simulink library "CellsLib"  (Simulink 7.7)
settings: Solver=ode45  SolverMode=SingleTasking  StartTime=0.0  StopTime=10.0  RelTol=1e-3
libraries: CompartmentsLib x26, CurrentsLib x23, SpikingLib x9, SynapsesLib x7, WaveformsLib x1, BasicSpikingElementsLib x1, SpikeToWavesLib x1, RateBasedLib x1
settings Model: Creator=jpalma  LastModifiedBy=jpalma

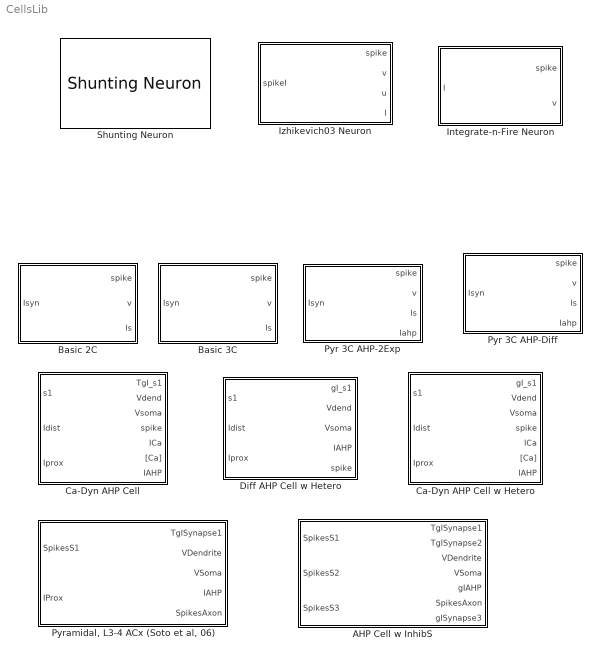
== system CellsLib ==
  AHP Cell w InhibS : Subsystem  mask{PSoma1=[1 -65 45 50 16 -100 0.1 -65 0.28 0.1 0.15], PDend2=[1 -65 0.03 -65 0.28 0.06 0.4], PDend3=[1 -65 0.03 -65 0.28 0.06 0.5], PfAHP=[-65 0.8 0.1 2.0], PmAHP=[-97 0.04 18 164], PsAHP=[-100 0.02 225 2200], PAmpa=[0 2 0.76 6.5], PAmpa2=[0 0.2 0.76 6.5], PGaba=[-90 2 0.76 6.5], spikeThreshold=10}
      mask prompts: PSoma1 "Soma Params [C1 V01 gNa1 ENa1 gK1 EK1 gL1 EL1 gA1 d1 L1]"; PDend2 "Prox Dend Params [C2 V02 gL2 EL2 gA2 d2 L2]"; PDend3 "Dist Dend Params [C3 V03 gL3 EL3 gA3 d3 L3]"; PfAHP "fAHP Params [EfAHP gfAHP RTfAHP FTfAHP]"; PmAHP "mAHP Params [EmAHP gmAHP RTmAHP FTmAHP]"; PsAHP "sAHP Params [EsAHP gsAHP RTsAHP FTsAHP]"; PAmpa "AMPA Params [EAmpa gAmpa RTampa FTampa]"; PAmpa2 "AMPA2 Params [EAmpa2 gAmpa2 RTampa2 FTampa2]"; PGaba "GABA Params [EGaba gGaba RTgaba FTgaba]"; spikeThreshold "Spike Detection Voltage Threshold"
      mask help: Author: Jesse Palma
      mask Help: Author: Jesse Palma
      mask Display: image(imread('../Libs/icons/Cell.jpg'),'center');
  Basic 2C : Subsystem  mask{PSoma1=[1 -65 45 50 16 -100 0.1 -65 0.28 0.1 0.15], PDend2=[1 -65 0.03 -65 0.28 0.06 0.4], spikeThreshold=10}
      mask prompts: PSoma1 "Soma Params [C1 V01 gNa1 ENa1 gK1 EK1 gL1 EL1 gA1 d1 L1]"; PDend2 "Dend Params [C2 V02 gL2 EL2 gA2 d2 L2]"; spikeThreshold "Spike Detection Voltage Threshold"
      mask help: Author: Jesse Palma
      settings: AttributesFormatString=%<AncestorBlock>
      mask Help: Author: Jesse Palma
      mask Display: image(imread('../Libs/icons/Cell.jpg'),'center');
  Basic 3C : Subsystem  mask{PSoma1=[1 -65 45 50 16 -100 0.1 -65 0.28 0.1 0.15], PDend2=[1 -65 0.03 -65 0.28 0.06 0.4], PDend3=[1 -65 0.03 -65 0.28 0.06 0.5], spikeThreshold=10}
      mask prompts: PSoma1 "Soma Params [C1 V01 gNa1 ENa1 gK1 EK1 gL1 EL1 gA1 d1 L1]"; PDend2 "Prox Dend Params [C2 V02 gL2 EL2 gA2 d2 L2]"; PDend3 "Dist Dend Params [C3 V03 gL3 EL3 gA3 d3 L3]"; spikeThreshold "Spike Detection Voltage Threshold"
      mask help: Author: Jesse Palma
      settings: AttributesFormatString=%<AncestorBlock>
      mask Help: Author: Jesse Palma
      mask Display: image(imread('../Libs/icons/Cell.jpg'),'center');
  Ca-Dyn AHP Cell : Subsystem  mask{C1=1, V01=-65, spikeThreshold=10, gA1=0.28, d1=0.1, L1=0.15, gNa1=45, ENa1=50, gK1=16, EK1=-100, gL1=0.1, EL1=-65, gBK1=4.0, EBK1=-65, gKA=0.5, EKA=-100, gSK1=0.08, ESK1=-97, gKM=0.1, EKM=-97, gsAHP1=0.025, EsAHP1=-100, gvsAHP=0.1, EvsAHP=-100, C2=1, V02=-65, gL2=0.03, EL2=-65, gA2=0.28, d2=0.06, L2=0.4, C3=1, V03=-65, gL3=0.03, EL3=-65, gA3=0.28, d3=0.06, L3=0.5, gampa=1, Eampa=0, RTampa=0.76, FTampa=6.5}
      mask prompts: C1 "Capacitance"; V01 "Initial Voltage"; spikeThreshold "Spike Detection Voltage Threshold"; gA1 "Axial Conductance"; d1 "Diameter"; L1 "Length"; gNa1 "Sodium Conductance"; ENa1 "Sodium Equilibrium Potential"; gK1 "Potassium Conductance"; EK1 "Potassium Equilibrium Potential"; gL1 "Leak Conductance"; EL1 "Leak Equilibrium Potential"; gBK1 "BK Conductance"; EBK1 "BK Equilibrium Potential"; gKA "K(A) Conductance"; EKA "K(A) Equilibrium Potential"; gSK1 "SK Conductance"; ESK1 "SK Equilibrium Potential"; gKM "K(M) Conductance"; EKM "K(M) Equilibrium Potential"; gsAHP1 "sAHP Conductance"; EsAHP1 "sAHP Equilibrium Potential"; gvsAHP "V sAHP Conductance"; EvsAHP "V sAHP Equilibrium Potential"; C2 "Capacitance"; V02 "Initial Voltage"; gL2 "Leak Conductance"; EL2 "Leak Equilibrium Potential"; gA2 "Axial Conductance"; d2 "Diameter"; L2 "Length"; C3 "Capacitance"; V03 "Initial Voltage"; gL3 "Leak Conductance"; EL3 "Leak Equilibrium Potential"; gA3 "Axial Conductance"; d3 "Diameter"; L3 "Length"; gampa "Conductance"; Eampa "Equilibrium Potential"; RTampa "Rise Time"; FTampa "Fall Time"
      mask help: Author: Jesse Palma
      mask Help: Author: Jesse Palma
      mask TabNameString: Soma Base, Soma Base, Soma Base, Soma Base, Soma Base, Soma Base,Currents,Currents,Currents,Currents,Currents,Currents,AHP,AHP,AHP,AHP,AHP,AHP,AHP,AHP,AHP,AHP,AHP,AHP,Prox,Prox,Prox,Prox,Prox,Prox,Prox,Dist,Dist,Dist,Dist,Dist,Dist,Dist,AMPA,AMPA,AMPA,AMPA
      mask Display: image(imread('../Libs/icons/Cell.jpg'),'center');
  Ca-Dyn AHP Cell w Hetero : Subsystem  mask{C1=1, V01=-65, spikeThreshold=10, gA1=0.28, d1=0.1, L1=0.15, gNa1=45, ENa1=50, gK1=16, EK1=-100, gL1=0.1, EL1=-65, gBK1=4.0, EBK1=-65, gKA=0.5, EKA=-100, gSK1=0.08, ESK1=-97, gKM=0.1, EKM=-97, gsAHP1=0.025, EsAHP1=-100, gvsAHP=0.1, EvsAHP=-100, C2=1, V02=-65, gL2=0.03, EL2=-65, gA2=0.28, d2=0.06, L2=0.4, C3=1, V03=-65, gL3=0.03, EL3=-65, gA3=0.28, d3=0.06, L3=0.5, gampa=1, Eampa=0, RTampa=0.76, FTampa=6.5}
      mask prompts: C1 "Capacitance"; V01 "Initial Voltage"; spikeThreshold "Spike Detection Voltage Threshold"; gA1 "Axial Conductance"; d1 "Diameter"; L1 "Length"; gNa1 "Sodium Conductance"; ENa1 "Sodium Equilibrium Potential"; gK1 "Potassium Conductance"; EK1 "Potassium Equilibrium Potential"; gL1 "Leak Conductance"; EL1 "Leak Equilibrium Potential"; gBK1 "BK Conductance"; EBK1 "BK Equilibrium Potential"; gKA "K(A) Conductance"; EKA "K(A) Equilibrium Potential"; gSK1 "SK Conductance"; ESK1 "SK Equilibrium Potential"; gKM "K(M) Conductance"; EKM "K(M) Equilibrium Potential"; gsAHP1 "sAHP Conductance"; EsAHP1 "sAHP Equilibrium Potential"; gvsAHP "V sAHP Conductance"; EvsAHP "V sAHP Equilibrium Potential"; C2 "Capacitance"; V02 "Initial Voltage"; gL2 "Leak Conductance"; EL2 "Leak Equilibrium Potential"; gA2 "Axial Conductance"; d2 "Diameter"; L2 "Length"; C3 "Capacitance"; V03 "Initial Voltage"; gL3 "Leak Conductance"; EL3 "Leak Equilibrium Potential"; gA3 "Axial Conductance"; d3 "Diameter"; L3 "Length"; gampa "Conductance"; Eampa "Equilibrium Potential"; RTampa "Rise Time"; FTampa "Fall Time"
      mask help: Author: Jesse Palma
      mask Help: Author: Jesse Palma
      mask TabNameString: Soma Base, Soma Base, Soma Base, Soma Base, Soma Base, Soma Base,Currents,Currents,Currents,Currents,Currents,Currents,AHP,AHP,AHP,AHP,AHP,AHP,AHP,AHP,AHP,AHP,AHP,AHP,Prox,Prox,Prox,Prox,Prox,Prox,Prox,Dist,Dist,Dist,Dist,Dist,Dist,Dist,AMPA,AMPA,AMPA,AMPA
      mask Display: image(imread('../Libs/icons/Cell.jpg'),'center');
  "Diff AHP Cell w Hetero " : Subsystem  mask{PSoma1=[1 -65 45 50 16 -100 0.1 -65 0.28 0.1 0.15], PDend2=[1 -65 0.03 -65 0.28 0.06 0.4], PDend3=[1 -65 0.03 -65 0.28 0.06 0.5], PfAHP=[-65 0.8 0.1 2.0], PmAHP=[-97 0.04 18 164], PsAHP=[-100 0.02 225 2200], PAmpa=[0 1 0.76 6.5], spikeThreshold=10}
      mask prompts: PSoma1 "Soma Params [C1 V01 gNa1 ENa1 gK1 EK1 gL1 EL1 gA1 d1 L1]"; PDend2 "Prox Dend Params [C2 V02 gL2 EL2 gA2 d2 L2]"; PDend3 "Dist Dend Params [C3 V03 gL3 EL3 gA3 d3 L3]"; PfAHP "fAHP Params [EfAHP gfAHP RTfAHP FTfAHP]"; PmAHP "mAHP Params [EmAHP gmAHP RTmAHP FTmAHP]"; PsAHP "sAHP Params [EsAHP gsAHP RTsAHP FTsAHP]"; PAmpa "AMPA Params [EAmpa gAmpa RTampa FTampa]"; spikeThreshold "Spike Detection Voltage Threshold"
      mask help: Author: Jesse Palma
      mask Help: Author: Jesse Palma
      mask Display: image(imread('../Libs/icons/Cell.jpg'),'center');
  Integrate-n-Fire Neuron : Subsystem  mask{A=0.05, SpikeThreshold=1}
      mask prompts: A "Decay Rate"; SpikeThreshold "Spike Threshold"
      mask help: Author: Jesse Palma
      mask Help: Author: Jesse Palma
      mask Display: image(imread('IntFire.JPG'),'center');
  Izhikevich03 Neuron : Subsystem
      mask Description: Author: Jesse Palma
      mask Help: Author: Jesse Palma
      mask Display: image(imread('../Libs/icons/Izhik.jpg'),'center');
  Pyr 3C AHP-2Exp : Subsystem  mask{PSoma1=[1 -65 45 50 16 -100 0.1 -65 0.28 0.1 0.15], PDend2=[1 -65 0.03 -65 0.28 0.06 0.4], PDend3=[1 -65 0.03 -65 0.28 0.06 0.5], PfAHP=[-65 0.8 0.1 2.0], PmAHP=[-97 0.04 18 164], PsAHP=[-100 0.02 225 2200], spikeThreshold=10}
      mask prompts: PSoma1 "Soma Params [C1 V01 gNa1 ENa1 gK1 EK1 gL1 EL1 gA1 d1 L1]"; PDend2 "Prox Dend Params [C2 V02 gL2 EL2 gA2 d2 L2]"; PDend3 "Dist Dend Params [C3 V03 gL3 EL3 gA3 d3 L3]"; PfAHP "fAHP Params [EfAHP gfAHP RTfAHP FTfAHP]"; PmAHP "mAHP Params [EmAHP gmAHP RTmAHP FTmAHP]"; PsAHP "sAHP Params [EsAHP gsAHP RTsAHP FTsAHP]"; spikeThreshold "Spike Detection Voltage Threshold"
      mask help: Author: Jesse Palma
      mask Help: Author: Jesse Palma
      mask Display: image(imread('../Libs/icons/Cell.jpg'),'center');
  Pyr 3C AHP-Diff : Subsystem  mask{PSoma1=[1 -65 45 50 16 -100 0.1 -65 0.28 0.1 0.15], PDend2=[1 -65 0.03 -65 0.28 0.06 0.4], PDend3=[1 -65 0.03 -65 0.28 0.06 0.5], PfAHP=[-65 0.8 0.1 2.0], PmAHP=[-97 0.04 18 164], PsAHP=[-100 0.02 225 2200], spikeThreshold=10}
      mask prompts: PSoma1 "Soma Params [C1 V01 gNa1 ENa1 gK1 EK1 gL1 EL1 gA1 d1 L1]"; PDend2 "Prox Dend Params [C2 V02 gL2 EL2 gA2 d2 L2]"; PDend3 "Dist Dend Params [C3 V03 gL3 EL3 gA3 d3 L3]"; PfAHP "fAHP Params [EfAHP gfAHP RTfAHP FTfAHP]"; PmAHP "mAHP Params [EmAHP gmAHP RTmAHP FTmAHP]"; PsAHP "sAHP Params [EsAHP gsAHP RTsAHP FTsAHP]"; spikeThreshold "Spike Detection Voltage Threshold"
      mask help: Author: Jesse Palma
      settings: AttributesFormatString=%<AncestorBlock>
      mask Help: Author: Jesse Palma
      mask Display: image(imread('../Libs/icons/Cell.jpg'),'center');
  "Pyramidal, L3-4 ACx (Soto et al, 06)" : Subsystem  mask{PSoma1=[1 -65 45 50 16 -100 0.1 -65 0.28 0.1 0.15], PDend2=[1 -65 0.03 -65 0.28 0.06 0.4], PDend3=[1 -65 0.03 -65 0.28 0.06 0.5], PfAHP=[-65 0.8 0.1 2.0], PmAHP=[-97 0.04 18 164], PsAHP=[-100 0.02 225 2200], PAmpa=[0 1 0.76 6.5], spikeThreshold=10}
      mask prompts: PSoma1 "Soma Params [C1 V01 gNa1 ENa1 gK1 EK1 gL1 EL1 gA1 d1 L1]"; PDend2 "Prox Dend Params [C2 V02 gL2 EL2 gA2 d2 L2]"; PDend3 "Dist Dend Params [C3 V03 gL3 EL3 gA3 d3 L3]"; PfAHP "fAHP Params [EfAHP gfAHP RTfAHP FTfAHP]"; PmAHP "mAHP Params [EmAHP gmAHP RTmAHP FTmAHP]"; PsAHP "sAHP Params [EsAHP gsAHP RTsAHP FTsAHP]"; PAmpa "AMPA Params [EAmpa gAmpa RTampa FTampa]"; spikeThreshold "Spike Detection Voltage Threshold"
      mask help: Author: Jesse Palma
      mask Help: Author: Jesse Palma
      mask Display: image(imread('../Libs/icons/Cell.jpg'),'center');
  Shunting Neuron : RateBasedLib/Shunting Neuron  SystemSampleTime=-1  A=0.1  B=1  tau=1

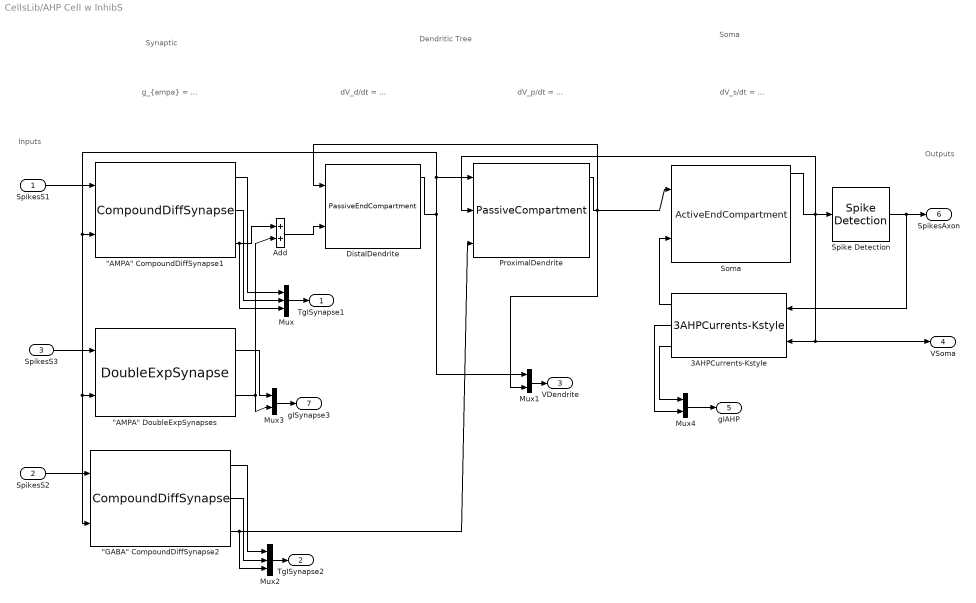
== system CellsLib/AHP Cell w InhibS ==
  note: Inputs
  note: Outputs
  note: Soma
  note: Dendritic Tree
  note: Synaptic
  note: g_{ampa} = ...
  note: dV_s/dt = ...
  note: dV_p/dt = ...
  note: dV_d/dt = ...
  SpikesS1 : Inport
  SpikesS2 : Inport  Port=2
  SpikesS3 : Inport  Port=3
  "\"AMPA\" CompoundDiffSynapse1" : SynapsesLib/CompoundDiffSynapse  SystemSampleTime=-1  EZ=PAmpa(1)  gZ=PAmpa(2)  tauRZ=PAmpa(3)  tauFZ=PAmpa(4)
  "\"AMPA\" DoubleExpSynapses" : SynapsesLib/DoubleExpSynapse  SystemSampleTime=-1  EZ=PAmpa2(1)  gZ=PAmpa2(2)  tauRZ=PAmpa2(3)  tauFZ=PAmpa2(4)
  "\"GABA\" CompoundDiffSynapse2" : SynapsesLib/CompoundDiffSynapse  SystemSampleTime=-1  EZ=PGaba(1)  gZ=PGaba(2)  tauRZ=PGaba(3)  tauFZ=PGaba(4)
  3AHPCurrents-Kstyle : CurrentsLib/3AHPCurrents-Kstyle  SystemSampleTime=-1  EfAHP=PfAHP(1)  gfAHP=PfAHP(2)  tauRfAHP=PfAHP(3)  tauFfAHP=PfAHP(4)  EmAHP=PmAHP(1)  gmAHP=PmAHP(2)  tauRmAHP=PmAHP(3)  tauFmAHP=PmAHP(4)  EsAHP=PsAHP(1)  gsAHP=PsAHP(2)  tauRsAHP=PsAHP(3)  tauFsAHP=PsAHP(4)
  Add : Sum
  DistalDendrite : CompartmentsLib/PassiveEndCompartment  SystemSampleTime=-1  C=PDend3(1)  V0=PDend3(2)  gA=PDend3(5)  d=PDend3(6)  L=PDend3(7)  gL=PDend3(3)  EL=PDend3(4)
  Mux : Mux  Inputs=3
  Mux1 : Mux  Inputs=2
  Mux2 : Mux  Inputs=3
  Mux3 : Mux  Inputs=2
  Mux4 : Mux  Inputs=2
  ProximalDendrite : CompartmentsLib/PassiveCompartment  SystemSampleTime=-1  C=PDend2(1)  V0=PDend2(2)  gA=PDend2(5)  d=PDend2(6)  L=PDend2(7)  gL=PDend2(3)  EL=PDend2(4)
  Soma : CompartmentsLib/ActiveEndCompartment  SystemSampleTime=-1  C=PSoma1(1)  V0=PSoma1(2)  gA=PSoma1(9)  d=PSoma1(10)  L=PSoma1(11)  gNa=PSoma1(3)  ENa=PSoma1(4)  gK=PSoma1(5)  EK=PSoma1(6)  gL=PSoma1(7)  EL=PSoma1(8)
  Spike Detection : SpikingLib/Spike Detection  SystemSampleTime=-1  SpikeVoltageThreshold=spikeThreshold
  TgISynapse1 : Outport
  TgISynapse2 : Outport  Port=2
  VDendrite : Outport  Port=3
  VSoma : Outport  Port=4
  gIAHP : Outport  Port=5
  SpikesAxon : Outport  Port=6
  gISynapse3 : Outport  Port=7
  wires:
  Mux1/1 -> VDendrite/1
  "\"AMPA\" CompoundDiffSynapse1"/1 -> Mux/1
  Mux/1 -> TgISynapse1/1
  "\"AMPA\" CompoundDiffSynapse1"/3 -> Mux/3, Add/1
  "\"AMPA\" CompoundDiffSynapse1"/2 -> Mux/2
  SpikesS1/1 -> "\"AMPA\" CompoundDiffSynapse1"/1
  Spike Detection/1 -> 3AHPCurrents-Kstyle/1, SpikesAxon/1
  Soma/1 -> ProximalDendrite/2, 3AHPCurrents-Kstyle/2, VSoma/1, Spike Detection/1
  ProximalDendrite/1 -> Mux1/2, Soma/1, DistalDendrite/1
  DistalDendrite/1 -> Mux1/1, ProximalDendrite/1, "\"AMPA\" CompoundDiffSynapse1"/2, "\"GABA\" CompoundDiffSynapse2"/2, "\"AMPA\" DoubleExpSynapses"/2
  SpikesS2/1 -> "\"GABA\" CompoundDiffSynapse2"/1
  Mux2/1 -> TgISynapse2/1
  "\"GABA\" CompoundDiffSynapse2"/1 -> Mux2/1
  "\"GABA\" CompoundDiffSynapse2"/2 -> Mux2/2
  "\"GABA\" CompoundDiffSynapse2"/3 -> ProximalDendrite/3, Mux2/3
  3AHPCurrents-Kstyle/1 -> Soma/2
  SpikesS3/1 -> "\"AMPA\" DoubleExpSynapses"/1
  Mux3/1 -> gISynapse3/1
  "\"AMPA\" DoubleExpSynapses"/1 -> Mux3/1
  "\"AMPA\" DoubleExpSynapses"/2 -> Mux3/2, Add/2
  Add/1 -> DistalDendrite/2
  Mux4/1 -> gIAHP/1
  3AHPCurrents-Kstyle/3 -> Mux4/1
  3AHPCurrents-Kstyle/2 -> Mux4/2

== system CellsLib/Basic 2C ==
  note: Soma
  note: dV_s/dt = ...
  note: dV_d/dt = ...
  note: Dendrite
  Isyn : Inport
  Bus Creator : BusCreator  Inputs=2
  Bus Creator1 : BusCreator
  Bus Selector : BusSelector  OutputSignals=signal1,signal2
  DistalDendrite : CompartmentsLib/PassiveEndCompartment  SystemSampleTime=-1  C=PDend2(1)  V0=PDend2(2)  gA=PDend2(5)  d=PDend2(6)  L=PDend2(7)  gL=PDend2(3)  EL=PDend2(4)
  Soma : CompartmentsLib/ActiveEndCompartment  SystemSampleTime=-1  C=PSoma1(1)  V0=PSoma1(2)  gA=PSoma1(9)  d=PSoma1(10)  L=PSoma1(11)  gNa=PSoma1(3)  ENa=PSoma1(4)  gK=PSoma1(5)  EK=PSoma1(6)  gL=PSoma1(7)  EL=PSoma1(8)
  Spike Detection : SpikingLib/Spike Detection  SystemSampleTime=-1  SpikeVoltageThreshold=spikeThreshold
  spike : Outport
  v : Outport  Port=2
  Is : Outport  Port=3
  wires:
  DistalDendrite/1 -> Soma/1, Bus Creator/1
  Soma/1 -> Spike Detection/1, DistalDendrite/1, Bus Creator/2
  Spike Detection/1 -> spike/1
  Isyn/1 -> Bus Selector/1
  Soma/2 -> Bus Creator1/1
  Soma/3 -> Bus Creator1/2
  Soma/4 -> Bus Creator1/3
  Soma/5 -> Bus Creator1/4
  Bus Creator1/1 -> Is/1
  Bus Selector/2 -> Soma/2
  Bus Creator/1 -> v/1
  Bus Selector/1 -> DistalDendrite/2

== system CellsLib/Basic 3C ==
  note: dV_d/dt = ...
  note: dV_p/dt = ...
  note: dV_s/dt = ...
  note: Dendritic Tree
  note: Soma
  Isyn : Inport
  Demux : Demux  Outputs=3
  DistalDendrite : CompartmentsLib/PassiveEndCompartment  SystemSampleTime=-1  C=PDend3(1)  V0=PDend3(2)  gA=PDend3(5)  d=PDend3(6)  L=PDend3(7)  gL=PDend3(3)  EL=PDend3(4)
  Mux : Mux
  Mux1 : Mux  Inputs=3
  ProximalDendrite : CompartmentsLib/PassiveCompartment  SystemSampleTime=-1  C=PDend2(1)  V0=PDend2(2)  gA=PDend2(5)  d=PDend2(6)  L=PDend2(7)  gL=PDend2(3)  EL=PDend2(4)
  Soma : CompartmentsLib/ActiveEndCompartment  SystemSampleTime=-1  C=PSoma1(1)  V0=PSoma1(2)  gA=PSoma1(9)  d=PSoma1(10)  L=PSoma1(11)  gNa=PSoma1(3)  ENa=PSoma1(4)  gK=PSoma1(5)  EK=PSoma1(6)  gL=PSoma1(7)  EL=PSoma1(8)
  Spike Detection : SpikingLib/Spike Detection  SystemSampleTime=-1  SpikeVoltageThreshold=spikeThreshold
  spike : Outport
  v : Outport  Port=2
  Is : Outport  Port=3
  wires:
  Mux1/1 -> v/1
  Demux/3 -> Soma/2
  Demux/2 -> ProximalDendrite/3
  Mux/1 -> Is/1
  Soma/5 -> Mux/4
  Soma/4 -> Mux/3
  Soma/3 -> Mux/2
  Soma/2 -> Mux/1
  Demux/1 -> DistalDendrite/2
  Isyn/1 -> Demux/1
  ProximalDendrite/1 -> Mux1/2, DistalDendrite/1, Soma/1
  Spike Detection/1 -> spike/1
  Soma/1 -> Mux1/3, ProximalDendrite/2, Spike Detection/1
  DistalDendrite/1 -> Mux1/1, ProximalDendrite/1

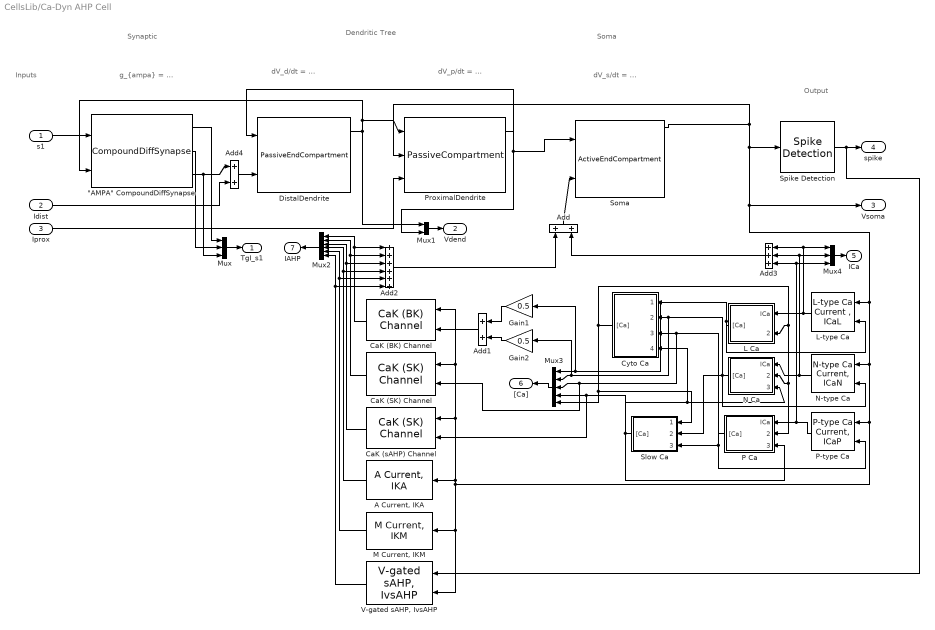
== system CellsLib/Ca-Dyn AHP Cell ==
  note: Inputs
  note: Output
  note: Soma
  note: Dendritic Tree
  note: Synaptic
  note: g_{ampa} = ...
  note: dV_s/dt = ...
  note: dV_p/dt = ...
  note: dV_d/dt = ...
  s1 : Inport
  Idist : Inport  Port=2
  Iprox : Inport  Port=3
  "\"AMPA\" CompoundDiffSynapse" : SynapsesLib/CompoundDiffSynapse  SystemSampleTime=-1  EZ=Eampa  gZ=gampa  tauRZ=RTampa  tauFZ=FTampa
  "A Current, IKA" : CurrentsLib/A Current, IKA  SystemSampleTime=-1  EKA=EKA  gKA=gKA  m_a=KAm_alpha  m_b=KAm_beta  h_a=KAh_alpha  h_b=KAh_beta
  Add : Sum
  Add1 : Sum
  Add2 : Sum  Inputs=++++++
  Add3 : Sum  Inputs=+++
  Add4 : Sum
  CaK (BK) Channel : CurrentsLib/CaK (BK) Channel  SystemSampleTime=-1  EBK=EBK1  gBK=gBK1
  CaK (SK) Channel : CurrentsLib/CaK (SK) Channel  SystemSampleTime=-1  ESK=ESK1  gSK=gSK1
  CaK (sAHP) Channel : CurrentsLib/CaK (SK) Channel  SystemSampleTime=-1  ESK=EsAHP1  gSK=gsAHP1
  Cyto Ca : Subsystem  mask{tauDiff1=800, tauDiff4=3600, tauA=80, caRest=1*10^(-6)}
      mask prompts: tauDiff1 "Diffusion Time Constant, tauDiff1"; tauDiff4 "Diffusion Time Constant, tauDiff4"; tauA "Recovery Time Constant, tauA"; caRest "Calcium Rest Concentration, caRest"
  DistalDendrite : CompartmentsLib/PassiveEndCompartment  SystemSampleTime=-1  C=C3  V0=V03  gA=gA3  d=d3  L=L3  gL=gL3  EL=EL3
  Gain1 : Gain  Gain=0.5
  Gain2 : Gain  Gain=0.5
  L Ca : Subsystem  mask{f=10000/(69843), d=800, a=1/120}
  L-type Ca : CurrentsLib/L-type Ca Current , ICaL  SystemSampleTime=-1  ECaL=130  gCaL=0.00006  m_e=caLm_infin2  m_t=cam_tau2  h_e=caLh_infin2  h_t=cah_tau2
  "M Current, IKM" : CurrentsLib/M Current, IKM  SystemSampleTime=-1  EK=EKM  gK=gKM  m_a=kMm_alpha  m_b=kMm_beta
  Mux : Mux  Inputs=3
  Mux1 : Mux  Inputs=2
  Mux2 : Mux  Inputs=6
  Mux3 : Mux  Inputs=5
  Mux4 : Mux  Inputs=3
  N Ca : Subsystem  mask{f=10000/(69843), d1=800, d2=3600, a=1/360}
  N-type Ca : CurrentsLib/N-type Ca Current, ICaN  SystemSampleTime=-1  ECaN=130  gCaN=0.00005  m_e=caNm_infin2  m_t=cam_tau2  h_e=caNh_infin2  h_t=cah_tau2
  P Ca : Subsystem  mask{f=10000/(69843), d1=800, d2=3600, a=1/60}
  P-type Ca : CurrentsLib/P-type Ca Current, ICaP  SystemSampleTime=-1  ECaP=130  gCaP=0.00009  m_e=caPm_infin2  m_t=cam_tau2  h_e=caPh_infin2  h_t=cah_tau2
  ProximalDendrite : CompartmentsLib/PassiveCompartment  SystemSampleTime=-1  C=C2  V0=V02  gA=gA2  d=d2  L=L2  gL=gL2  EL=EL2
  Slow Ca : Subsystem  mask{tauDiff1=3600, tauDiff2=3600, tauDiff3=3600}
      mask prompts: tauDiff1 "Diffusion Time Constant, tauDiff1"; tauDiff2 "Diffusion Time Constant, tauDiff2"; tauDiff3 "Diffusion Time Constant, tauDiff3"
  Soma : CompartmentsLib/ActiveEndCompartment  SystemSampleTime=-1  C=C1  V0=V01  gA=gA1  d=d1  L=L1  gNa=gNa1  ENa=ENa1  gK=gK1  EK=EK1  gL=gL1  EL=EL1
  Spike Detection : SpikingLib/Spike Detection  SystemSampleTime=-1  SpikeVoltageThreshold=spikeThreshold
  "V-gated sAHP, IvsAHP" : CurrentsLib/V-gated sAHP, IvsAHP  SystemSampleTime=-1  EvsAHP=EvsAHP  gvsAHP=gvsAHP  RvsAHP=225  FvsAHP=2400
  TgI_s1 : Outport
  Vdend : Outport  Port=2
  Vsoma : Outport  Port=3
  spike : Outport  Port=4
  ICa : Outport  Port=5
  "[Ca]" : Outport  Port=6
  IAHP : Outport  Port=7
  wires:
  Mux1/1 -> Vdend/1
  "\"AMPA\" CompoundDiffSynapse"/1 -> Mux/1
  Mux/1 -> TgI_s1/1
  "\"AMPA\" CompoundDiffSynapse"/3 -> Mux/3, Add4/1
  Iprox/1 -> ProximalDendrite/3
  "\"AMPA\" CompoundDiffSynapse"/2 -> Mux/2
  s1/1 -> "\"AMPA\" CompoundDiffSynapse"/1
  Spike Detection/1 -> spike/1, "V-gated sAHP, IvsAHP"/1
  ProximalDendrite/1 -> Mux1/2, Soma/1, DistalDendrite/1
  DistalDendrite/1 -> Mux1/1, ProximalDendrite/1, "\"AMPA\" CompoundDiffSynapse"/2
  L-type Ca/1 -> L Ca/1(ICa), Add3/1, Mux4/1
  P-type Ca/1 -> P Ca/1(ICa), Add3/3, Mux4/3
  L Ca/1("[Ca]") -> Mux3/1, Gain1/1, Cyto Ca/1(AdjCa1), L-type Ca/2
  N Ca/1("[Ca]") -> N-type Ca/2, Slow Ca/2(AdjCa2), Mux3/2, Gain2/1, Cyto Ca/2(AdjCa2)
  P Ca/1("[Ca]") -> P-type Ca/2, Slow Ca/3(AdjCa3), Cyto Ca/3(AdjCa3), Mux3/3, CaK (SK) Channel/2
  Mux3/1 -> "[Ca]"/1
  CaK (SK) Channel/1 -> Add2/2, Mux2/2
  CaK (sAHP) Channel/1 -> Add2/3, Mux2/3
  Soma/1 -> Vsoma/1, L-type Ca/1, N-type Ca/1, P-type Ca/1, CaK (BK) Channel/1, CaK (SK) Channel/1, CaK (sAHP) Channel/1, "V-gated sAHP, IvsAHP"/2, "M Current, IKM"/1, "A Current, IKA"/1, Spike Detection/1, ProximalDendrite/2
  Add/1 -> Soma/2
  Cyto Ca/1("[Ca]") -> L Ca/2(AdjCa), N Ca/2(AdjCa1), P Ca/2(AdjCa1), Slow Ca/1(AdjCa1), Mux3/5
  Slow Ca/1("[Ca]") -> Mux3/4, CaK (sAHP) Channel/2, P Ca/3(AdjCa2), N Ca/3(AdjCa2), Cyto Ca/4(AdjCa4)
  N-type Ca/1 -> N Ca/1(ICa), Add3/2, Mux4/2
  Gain1/1 -> Add1/1
  Gain2/1 -> Add1/2
  Add1/1 -> CaK (BK) Channel/2
  CaK (BK) Channel/1 -> Add2/1, Mux2/1
  Add2/1 -> Add/1
  Add3/1 -> Add/2
  Mux2/1 -> IAHP/1
  Mux4/1 -> ICa/1
  "A Current, IKA"/1 -> Add2/4, Mux2/4
  "M Current, IKM"/1 -> Add2/5, Mux2/5
  "V-gated sAHP, IvsAHP"/1 -> Mux2/6, Add2/6
  Add4/1 -> DistalDendrite/2
  Idist/1 -> Add4/2

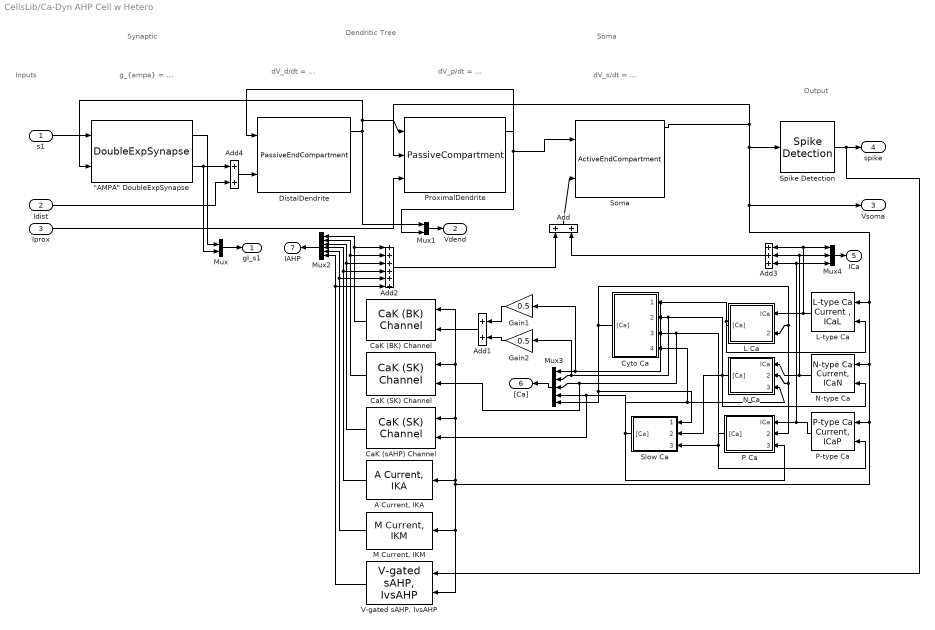
== system CellsLib/Ca-Dyn AHP Cell w Hetero ==
  note: dV_d/dt = ...
  note: dV_p/dt = ...
  note: dV_s/dt = ...
  note: g_{ampa} = ...
  note: Synaptic
  note: Dendritic Tree
  note: Soma
  note: Output
  note: Inputs
  s1 : Inport
  Idist : Inport  Port=2
  Iprox : Inport  Port=3
  "\"AMPA\" DoubleExpSynapse" : SynapsesLib/DoubleExpSynapse  SystemSampleTime=-1  EZ=Eampa  gZ=gampa  tauRZ=RTampa  tauFZ=FTampa
  "A Current, IKA" : CurrentsLib/A Current, IKA  SystemSampleTime=-1  EKA=EKA  gKA=gKA  m_a=KAm_alpha  m_b=KAm_beta  h_a=KAh_alpha  h_b=KAh_beta
  Add : Sum
  Add1 : Sum
  Add2 : Sum  Inputs=++++++
  Add3 : Sum  Inputs=+++
  Add4 : Sum
  CaK (BK) Channel : CurrentsLib/CaK (BK) Channel  SystemSampleTime=-1  EBK=EBK1  gBK=gBK1
  CaK (SK) Channel : CurrentsLib/CaK (SK) Channel  SystemSampleTime=-1  ESK=ESK1  gSK=gSK1
  CaK (sAHP) Channel : CurrentsLib/CaK (SK) Channel  SystemSampleTime=-1  ESK=EsAHP1  gSK=gsAHP1
  Cyto Ca : Subsystem  mask{tauDiff1=800, tauDiff4=3600, tauA=80, caRest=1*10^(-6)}
      mask prompts: tauDiff1 "Diffusion Time Constant, tauDiff1"; tauDiff4 "Diffusion Time Constant, tauDiff4"; tauA "Recovery Time Constant, tauA"; caRest "Calcium Rest Concentration, caRest"
  DistalDendrite : CompartmentsLib/PassiveEndCompartment  SystemSampleTime=-1  C=C3  V0=V03  gA=gA3  d=d3  L=L3  gL=gL3  EL=EL3
  Gain1 : Gain  Gain=0.5
  Gain2 : Gain  Gain=0.5
  L Ca : Subsystem  mask{f=10000/(69843), d=800, a=1/120}
  L-type Ca : CurrentsLib/L-type Ca Current , ICaL  SystemSampleTime=-1  ECaL=130  gCaL=0.00006  m_e=caLm_infin2  m_t=cam_tau2  h_e=caLh_infin2  h_t=cah_tau2
  "M Current, IKM" : CurrentsLib/M Current, IKM  SystemSampleTime=-1  EK=EKM  gK=gKM  m_a=kMm_alpha  m_b=kMm_beta
  Mux : Mux  Inputs=2
  Mux1 : Mux  Inputs=2
  Mux2 : Mux  Inputs=6
  Mux3 : Mux  Inputs=5
  Mux4 : Mux  Inputs=3
  N Ca : Subsystem  mask{f=10000/(69843), d1=800, d2=3600, a=1/360}
  N-type Ca : CurrentsLib/N-type Ca Current, ICaN  SystemSampleTime=-1  ECaN=130  gCaN=0.00005  m_e=caNm_infin2  m_t=cam_tau2  h_e=caNh_infin2  h_t=cah_tau2
  P Ca : Subsystem  mask{f=10000/(69843), d1=800, d2=3600, a=1/60}
  P-type Ca : CurrentsLib/P-type Ca Current, ICaP  SystemSampleTime=-1  ECaP=130  gCaP=0.00009  m_e=caPm_infin2  m_t=cam_tau2  h_e=caPh_infin2  h_t=cah_tau2
  ProximalDendrite : CompartmentsLib/PassiveCompartment  SystemSampleTime=-1  C=C2  V0=V02  gA=gA2  d=d2  L=L2  gL=gL2  EL=EL2
  Slow Ca : Subsystem  mask{tauDiff1=3600, tauDiff2=3600, tauDiff3=3600}
      mask prompts: tauDiff1 "Diffusion Time Constant, tauDiff1"; tauDiff2 "Diffusion Time Constant, tauDiff2"; tauDiff3 "Diffusion Time Constant, tauDiff3"
  Soma : CompartmentsLib/ActiveEndCompartment  SystemSampleTime=-1  C=C1  V0=V01  gA=gA1  d=d1  L=L1  gNa=gNa1  ENa=ENa1  gK=gK1  EK=EK1  gL=gL1  EL=EL1
  Spike Detection : SpikingLib/Spike Detection  SystemSampleTime=-1  SpikeVoltageThreshold=spikeThreshold
  "V-gated sAHP, IvsAHP" : CurrentsLib/V-gated sAHP, IvsAHP  SystemSampleTime=-1  EvsAHP=EvsAHP  gvsAHP=gvsAHP  RvsAHP=225  FvsAHP=2400
  gI_s1 : Outport
  Vdend : Outport  Port=2
  Vsoma : Outport  Port=3
  spike : Outport  Port=4
  ICa : Outport  Port=5
  "[Ca]" : Outport  Port=6
  IAHP : Outport  Port=7
  wires:
  Idist/1 -> Add4/2
  Add4/1 -> DistalDendrite/2
  "V-gated sAHP, IvsAHP"/1 -> Add2/6, Mux2/6
  "M Current, IKM"/1 -> Mux2/5, Add2/5
  "A Current, IKA"/1 -> Mux2/4, Add2/4
  Mux4/1 -> ICa/1
  Mux2/1 -> IAHP/1
  Add3/1 -> Add/2
  Add2/1 -> Add/1
  CaK (BK) Channel/1 -> Mux2/1, Add2/1
  Add1/1 -> CaK (BK) Channel/2
  Gain2/1 -> Add1/2
  Gain1/1 -> Add1/1
  N-type Ca/1 -> Mux4/2, Add3/2, N Ca/1(ICa)
  Slow Ca/1("[Ca]") -> Cyto Ca/4(AdjCa4), N Ca/3(AdjCa2), P Ca/3(AdjCa2), CaK (sAHP) Channel/2, Mux3/4
  Cyto Ca/1("[Ca]") -> Mux3/5, Slow Ca/1(AdjCa1), P Ca/2(AdjCa1), N Ca/2(AdjCa1), L Ca/2(AdjCa)
  Add/1 -> Soma/2
  Soma/1 -> ProximalDendrite/2, Spike Detection/1, "A Current, IKA"/1, "M Current, IKM"/1, "V-gated sAHP, IvsAHP"/2, CaK (sAHP) Channel/1, CaK (SK) Channel/1, CaK (BK) Channel/1, P-type Ca/1, N-type Ca/1, L-type Ca/1, Vsoma/1
  CaK (sAHP) Channel/1 -> Mux2/3, Add2/3
  CaK (SK) Channel/1 -> Mux2/2, Add2/2
  Mux3/1 -> "[Ca]"/1
  P Ca/1("[Ca]") -> CaK (SK) Channel/2, Mux3/3, Cyto Ca/3(AdjCa3), Slow Ca/3(AdjCa3), P-type Ca/2
  N Ca/1("[Ca]") -> Cyto Ca/2(AdjCa2), Gain2/1, Mux3/2, Slow Ca/2(AdjCa2), N-type Ca/2
  L Ca/1("[Ca]") -> L-type Ca/2, Cyto Ca/1(AdjCa1), Gain1/1, Mux3/1
  P-type Ca/1 -> Mux4/3, Add3/3, P Ca/1(ICa)
  L-type Ca/1 -> Mux4/1, Add3/1, L Ca/1(ICa)
  DistalDendrite/1 -> ProximalDendrite/1, "\"AMPA\" DoubleExpSynapse"/2, Mux1/1
  ProximalDendrite/1 -> DistalDendrite/1, Soma/1, Mux1/2
  Spike Detection/1 -> "V-gated sAHP, IvsAHP"/1, spike/1
  s1/1 -> "\"AMPA\" DoubleExpSynapse"/1
  Iprox/1 -> ProximalDendrite/3
  "\"AMPA\" DoubleExpSynapse"/2 -> Add4/1, Mux/2
  Mux/1 -> gI_s1/1
  Mux1/1 -> Vdend/1
  "\"AMPA\" DoubleExpSynapse"/1 -> Mux/1

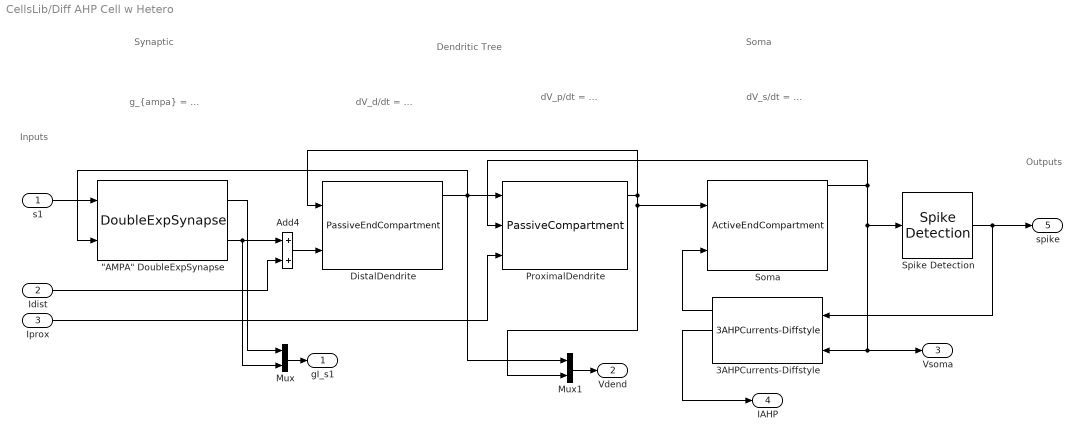
== system CellsLib/Diff AHP Cell w Hetero  ==
  note: dV_d/dt = ...
  note: dV_p/dt = ...
  note: dV_s/dt = ...
  note: g_{ampa} = ...
  note: Synaptic
  note: Dendritic Tree
  note: Soma
  note: Outputs
  note: Inputs
  s1 : Inport
  Idist : Inport  Port=2
  Iprox : Inport  Port=3
  "\"AMPA\" DoubleExpSynapse" : SynapsesLib/DoubleExpSynapse  SystemSampleTime=-1  EZ=PAmpa(1)  gZ=PAmpa(2)  tauRZ=PAmpa(3)  tauFZ=PAmpa(4)
  3AHPCurrents-Diffstyle : CurrentsLib/3AHPCurrents-Diffstyle  SystemSampleTime=-1  EfAHP=PfAHP(1)  gfAHP=PfAHP(2)  tauRfAHP=PfAHP(3)  tauFfAHP=PfAHP(4)  EmAHP=PmAHP(1)  gmAHP=PmAHP(2)  tauRmAHP=PmAHP(3)  tauFmAHP=PmAHP(4)  EsAHP=PsAHP(1)  gsAHP=PsAHP(2)  tauRsAHP=PsAHP(3)  tauFsAHP=PsAHP(4)
  Add4 : Sum
  DistalDendrite : CompartmentsLib/PassiveEndCompartment  SystemSampleTime=-1  C=PDend3(1)  V0=PDend3(2)  gA=PDend3(5)  d=PDend3(6)  L=PDend3(7)  gL=PDend3(3)  EL=PDend3(4)
  Mux : Mux  Inputs=2
  Mux1 : Mux  Inputs=2
  ProximalDendrite : CompartmentsLib/PassiveCompartment  SystemSampleTime=-1  C=PDend2(1)  V0=PDend2(2)  gA=PDend2(5)  d=PDend2(6)  L=PDend2(7)  gL=PDend2(3)  EL=PDend2(4)
  Soma : CompartmentsLib/ActiveEndCompartment  SystemSampleTime=-1  C=PSoma1(1)  V0=PSoma1(2)  gA=PSoma1(9)  d=PSoma1(10)  L=PSoma1(11)  gNa=PSoma1(3)  ENa=PSoma1(4)  gK=PSoma1(5)  EK=PSoma1(6)  gL=PSoma1(7)  EL=PSoma1(8)
  Spike Detection : SpikingLib/Spike Detection  SystemSampleTime=-1  SpikeVoltageThreshold=spikeThreshold
  gI_s1 : Outport
  Vdend : Outport  Port=2
  Vsoma : Outport  Port=3
  IAHP : Outport  Port=4
  spike : Outport  Port=5
  wires:
  Idist/1 -> Add4/2
  Add4/1 -> DistalDendrite/2
  ProximalDendrite/1 -> DistalDendrite/1, Soma/1, Mux1/2
  Spike Detection/1 -> 3AHPCurrents-Diffstyle/1, spike/1
  s1/1 -> "\"AMPA\" DoubleExpSynapse"/1
  Iprox/1 -> ProximalDendrite/3
  "\"AMPA\" DoubleExpSynapse"/2 -> Add4/1, Mux/2
  Mux/1 -> gI_s1/1
  Mux1/1 -> Vdend/1
  3AHPCurrents-Diffstyle/1 -> Soma/2
  Soma/1 -> ProximalDendrite/2, 3AHPCurrents-Diffstyle/2, Vsoma/1, Spike Detection/1
  DistalDendrite/1 -> ProximalDendrite/1, Mux1/1, "\"AMPA\" DoubleExpSynapse"/2
  3AHPCurrents-Diffstyle/2 -> IAHP/1
  "\"AMPA\" DoubleExpSynapse"/1 -> Mux/1

== system CellsLib/Integrate-n-Fire Neuron ==
  I : Inport
  Leaky Integrator w Reset : WaveformsLib/Leaky Integrator w Reset  SystemSampleTime=-1  X0=0  A=A
  Memory : Memory
  Spike Detection : HitCross  HitCrossingOffset=SpikeThreshold  HitCrossingDirection=rising
  spike : Outport
  v : Outport  Port=2
  wires:
  I/1 -> Leaky Integrator w Reset/1
  Spike Detection/1 -> spike/1, Memory/1
  Leaky Integrator w Reset/1 -> Spike Detection/1, v/1
  Memory/1 -> Leaky Integrator w Reset/2

== system CellsLib/Izhikevich03 Neuron ==
  spikeI : Inport
  Izhikevich 2003 : CompartmentsLib/Izhikevich 2003  SystemSampleTime=-1  settings=UserDefined  A=0.02  B=0.2  C=-65  D=8  P2=0.04  P1=5  P0=140  VP=30  V0=-70  U0=-20
  Spike Detection : BasicSpikingElementsLib/Spike Detection  SystemSampleTime=-1  SpikeVoltageThreshold=30
  Spike to Leaky Integrator : SpikeToWavesLib/Spike to Leaky Integrator  SystemSampleTime=-1  tauFall=20
  spike : Outport
  v : Outport  Port=2
  u : Outport  Port=3
  I : Outport  Port=4
  wires:
  Izhikevich 2003/2 -> u/1
  Spike to Leaky Integrator/1 -> I/1, Izhikevich 2003/1
  Izhikevich 2003/1 -> v/1, Spike Detection/1
  Spike Detection/1 -> spike/1
  spikeI/1 -> Spike to Leaky Integrator/1

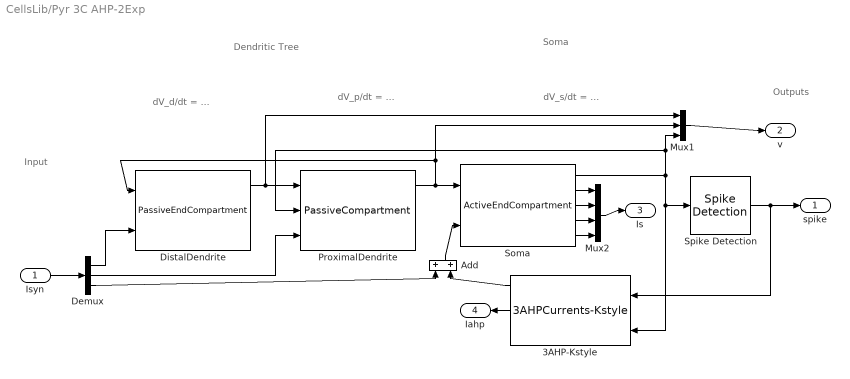
== system CellsLib/Pyr 3C AHP-2Exp ==
  note: dV_d/dt = ...
  note: dV_p/dt = ...
  note: dV_s/dt = ...
  note: Dendritic Tree
  note: Soma
  note: Outputs
  note: Input
  Isyn : Inport
  3AHP-Kstyle : CurrentsLib/3AHPCurrents-Kstyle  SystemSampleTime=-1  EfAHP=PfAHP(1)  gfAHP=PfAHP(2)  tauRfAHP=PfAHP(3)  tauFfAHP=PfAHP(4)  EmAHP=PmAHP(1)  gmAHP=PmAHP(2)  tauRmAHP=PmAHP(3)  tauFmAHP=PmAHP(4)  EsAHP=PsAHP(1)  gsAHP=PsAHP(2)  tauRsAHP=PsAHP(3)  tauFsAHP=PsAHP(4)
  Add : Sum
  Demux : Demux  Outputs=3
  DistalDendrite : CompartmentsLib/PassiveEndCompartment  SystemSampleTime=-1  C=PDend3(1)  V0=PDend3(2)  gA=PDend3(5)  d=PDend3(6)  L=PDend3(7)  gL=PDend3(3)  EL=PDend3(4)
  Mux1 : Mux  Inputs=3
  Mux2 : Mux
  ProximalDendrite : CompartmentsLib/PassiveCompartment  SystemSampleTime=-1  C=PDend2(1)  V0=PDend2(2)  gA=PDend2(5)  d=PDend2(6)  L=PDend2(7)  gL=PDend2(3)  EL=PDend2(4)
  Soma : CompartmentsLib/ActiveEndCompartment  SystemSampleTime=-1  C=PSoma1(1)  V0=PSoma1(2)  gA=PSoma1(9)  d=PSoma1(10)  L=PSoma1(11)  gNa=PSoma1(3)  ENa=PSoma1(4)  gK=PSoma1(5)  EK=PSoma1(6)  gL=PSoma1(7)  EL=PSoma1(8)
  Spike Detection : SpikingLib/Spike Detection  SystemSampleTime=-1  SpikeVoltageThreshold=spikeThreshold
  spike : Outport
  v : Outport  Port=2
  Is : Outport  Port=3
  Iahp : Outport  Port=4
  wires:
  ProximalDendrite/1 -> Soma/1, DistalDendrite/1, Mux1/2
  Spike Detection/1 -> 3AHP-Kstyle/1, spike/1
  Soma/1 -> Spike Detection/1, 3AHP-Kstyle/2, ProximalDendrite/2, Mux1/3
  DistalDendrite/1 -> ProximalDendrite/1, Mux1/1
  Demux/1 -> DistalDendrite/2
  Demux/2 -> ProximalDendrite/3
  Mux1/1 -> v/1
  Add/1 -> Soma/2
  Demux/3 -> Add/1
  3AHP-Kstyle/1 -> Add/2
  Isyn/1 -> Demux/1
  Soma/2 -> Mux2/1
  Soma/3 -> Mux2/2
  Soma/4 -> Mux2/3
  Soma/5 -> Mux2/4
  Mux2/1 -> Is/1
  3AHP-Kstyle/2 -> Iahp/1

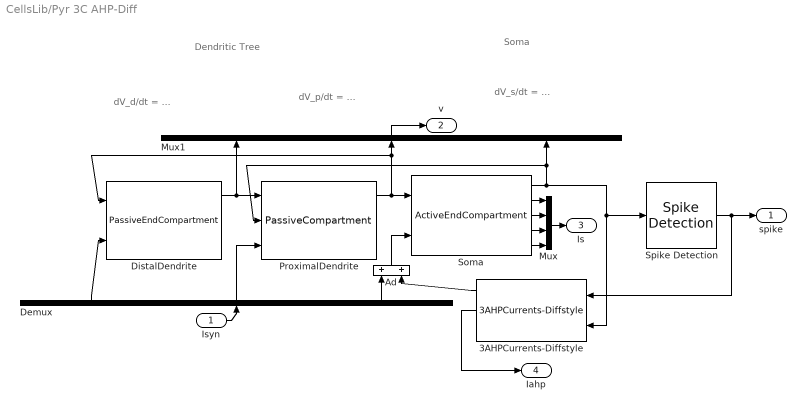
== system CellsLib/Pyr 3C AHP-Diff ==
  note: Soma
  note: Dendritic Tree
  note: dV_s/dt = ...
  note: dV_p/dt = ...
  note: dV_d/dt = ...
  Isyn : Inport
  3AHPCurrents-Diffstyle : CurrentsLib/3AHPCurrents-Diffstyle  SystemSampleTime=-1  EfAHP=PfAHP(1)  gfAHP=PfAHP(2)  tauRfAHP=PfAHP(3)  tauFfAHP=PfAHP(4)  EmAHP=PmAHP(1)  gmAHP=PmAHP(2)  tauRmAHP=PmAHP(3)  tauFmAHP=PmAHP(4)  EsAHP=PsAHP(1)  gsAHP=PsAHP(2)  tauRsAHP=PsAHP(3)  tauFsAHP=PsAHP(4)
  Ad : Sum
  Demux : Demux  Outputs=3
  DistalDendrite : CompartmentsLib/PassiveEndCompartment  SystemSampleTime=-1  C=PDend3(1)  V0=PDend3(2)  gA=PDend3(5)  d=PDend3(6)  L=PDend3(7)  gL=PDend3(3)  EL=PDend3(4)
  Mux : Mux
  Mux1 : Mux  Inputs=3
  ProximalDendrite : CompartmentsLib/PassiveCompartment  SystemSampleTime=-1  C=PDend2(1)  V0=PDend2(2)  gA=PDend2(5)  d=PDend2(6)  L=PDend2(7)  gL=PDend2(3)  EL=PDend2(4)
  Soma : CompartmentsLib/ActiveEndCompartment  SystemSampleTime=-1  C=PSoma1(1)  V0=PSoma1(2)  gA=PSoma1(9)  d=PSoma1(10)  L=PSoma1(11)  gNa=PSoma1(3)  ENa=PSoma1(4)  gK=PSoma1(5)  EK=PSoma1(6)  gL=PSoma1(7)  EL=PSoma1(8)
  Spike Detection : SpikingLib/Spike Detection  SystemSampleTime=-1  SpikeVoltageThreshold=spikeThreshold
  spike : Outport
  v : Outport  Port=2
  Is : Outport  Port=3
  Iahp : Outport  Port=4
  wires:
  3AHPCurrents-Diffstyle/2 -> Iahp/1
  DistalDendrite/1 -> ProximalDendrite/1, Mux1/1
  Soma/1 -> ProximalDendrite/2, Mux1/3, 3AHPCurrents-Diffstyle/2, Spike Detection/1
  Spike Detection/1 -> 3AHPCurrents-Diffstyle/1, spike/1
  ProximalDendrite/1 -> Soma/1, DistalDendrite/1, Mux1/2
  Isyn/1 -> Demux/1
  Demux/1 -> DistalDendrite/2
  Soma/2 -> Mux/1
  Soma/3 -> Mux/2
  Soma/4 -> Mux/3
  Soma/5 -> Mux/4
  Mux/1 -> Is/1
  Demux/2 -> ProximalDendrite/3
  Demux/3 -> Ad/1
  Ad/1 -> Soma/2
  3AHPCurrents-Diffstyle/1 -> Ad/2
  Mux1/1 -> v/1

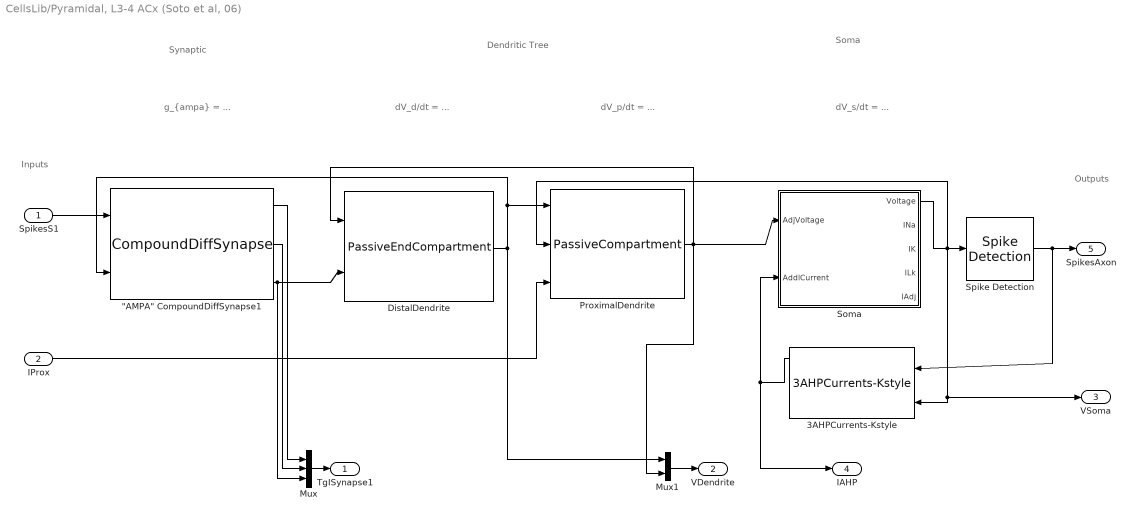
== system CellsLib/Pyramidal, L3-4 ACx (Soto et al, 06) ==
  note: Inputs
  note: Outputs
  note: Soma
  note: Dendritic Tree
  note: Synaptic
  note: g_{ampa} = ...
  note: dV_s/dt = ...
  note: dV_p/dt = ...
  note: dV_d/dt = ...
  SpikesS1 : Inport
  IProx : Inport  Port=2
  "\"AMPA\" CompoundDiffSynapse1" : SynapsesLib/CompoundDiffSynapse  SystemSampleTime=-1  EZ=PAmpa(1)  gZ=PAmpa(2)  tauRZ=PAmpa(3)  tauFZ=PAmpa(4)
  3AHPCurrents-Kstyle : CurrentsLib/3AHPCurrents-Kstyle  SystemSampleTime=-1  EfAHP=PfAHP(1)  gfAHP=PfAHP(2)  tauRfAHP=PfAHP(3)  tauFfAHP=PfAHP(4)  EmAHP=PmAHP(1)  gmAHP=PmAHP(2)  tauRmAHP=PmAHP(3)  tauFmAHP=PmAHP(4)  EsAHP=PsAHP(1)  gsAHP=PsAHP(2)  tauRsAHP=PsAHP(3)  tauFsAHP=PsAHP(4)
  DistalDendrite : CompartmentsLib/PassiveEndCompartment  SystemSampleTime=-1  C=PDend3(1)  V0=PDend3(2)  gL=PDend3(3)  EL=PDend3(4)  gA=PDend3(5)  d=PDend3(6)  L=PDend3(7)
  Mux : Mux  Inputs=3
  Mux1 : Mux  Inputs=2
  ProximalDendrite : CompartmentsLib/PassiveCompartment  SystemSampleTime=-1  C=PDend2(1)  V0=PDend2(2)  gL=PDend2(3)  EL=PDend2(4)  gA=PDend2(5)  d=PDend2(6)  L=PDend2(7)
  Soma : Subsystem  mask{C=PSoma1(1), V0=PSoma1(2), gNa=PSoma1(3), ENa=PSoma1(4), gK=PSoma1(5), EK=PSoma1(6), gL=PSoma1(7), EL=PSoma1(8), gA=PSoma1(9), d=PSoma1(10), L=PSoma1(11)}
      mask prompts: C "Capacitance, C"; V0 "Initial Voltage, V0"; gNa "Na Conductance, gNa"; ENa "Na Eq Voltage, ENa"; gK "K Conductance, gK"; EK "K Eq Voltage, EK"; gL "Leak Conductance, gL"; EL "Leak Eq Voltage, EL"; gA "Axial Conductance, gA"; d "Comp Diameter, d"; L "Comp Length, L"
      mask help: Author: Jesse Palma
      mask Help: Author: Jesse Palma
      mask Display: image(imread('..\Libs\icons\Compartment.jpg'),'center');
  Spike Detection : SpikingLib/Spike Detection  SystemSampleTime=-1  SpikeVoltageThreshold=spikeThreshold
  TgISynapse1 : Outport
  VDendrite : Outport  Port=2
  VSoma : Outport  Port=3
  IAHP : Outport  Port=4
  SpikesAxon : Outport  Port=5
  wires:
  Mux1/1 -> VDendrite/1
  3AHPCurrents-Kstyle/1 -> IAHP/1, Soma/2(AddlCurrent)
  "\"AMPA\" CompoundDiffSynapse1"/1 -> Mux/1
  Mux/1 -> TgISynapse1/1
  "\"AMPA\" CompoundDiffSynapse1"/3 -> Mux/3, DistalDendrite/2
  IProx/1 -> ProximalDendrite/3
  "\"AMPA\" CompoundDiffSynapse1"/2 -> Mux/2
  SpikesS1/1 -> "\"AMPA\" CompoundDiffSynapse1"/1
  Spike Detection/1 -> 3AHPCurrents-Kstyle/1, SpikesAxon/1
  Soma/1(Voltage) -> ProximalDendrite/2, 3AHPCurrents-Kstyle/2, VSoma/1, Spike Detection/1
  ProximalDendrite/1 -> Mux1/2, Soma/1(AdjVoltage), DistalDendrite/1
  DistalDendrite/1 -> Mux1/1, ProximalDendrite/1, "\"AMPA\" CompoundDiffSynapse1"/2

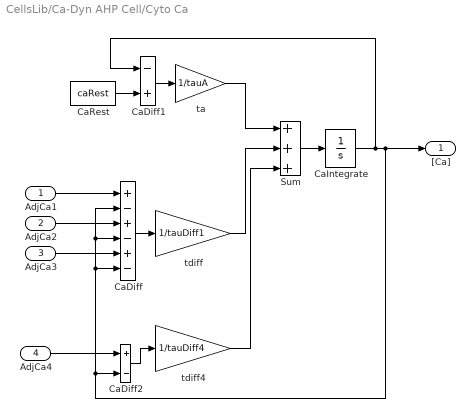
== system CellsLib/Ca-Dyn AHP Cell/Cyto Ca ==
  AdjCa1 : Inport
  AdjCa2 : Inport  Port=2
  AdjCa3 : Inport  Port=3
  AdjCa4 : Inport  Port=4
  CaDiff : Sum  Inputs=+-+-+-
  CaDiff1 : Sum  Inputs=-+
  CaDiff2 : Sum  Inputs=+-
  CaIntegrate : Integrator  InitialCondition=caRest
  CaRest : Constant  Value=caRest
  Sum : Sum  Inputs=+++
  ta : Gain  Gain=1/tauA
  tdiff : Gain  Gain=1/tauDiff1
  tdiff4 : Gain  Gain=1/tauDiff4
  "[Ca]" : Outport
  wires:
  tdiff/1 -> Sum/2
  CaDiff/1 -> tdiff/1
  CaIntegrate/1 -> CaDiff1/1, "[Ca]"/1, CaDiff2/2, CaDiff/6, CaDiff/4, CaDiff/2
  Sum/1 -> CaIntegrate/1
  CaRest/1 -> CaDiff1/2
  CaDiff1/1 -> ta/1
  ta/1 -> Sum/1
  AdjCa1/1 -> CaDiff/1
  AdjCa2/1 -> CaDiff/3
  AdjCa3/1 -> CaDiff/5
  CaDiff2/1 -> tdiff4/1
  tdiff4/1 -> Sum/3
  AdjCa4/1 -> CaDiff2/1

== system CellsLib/Ca-Dyn AHP Cell/L Ca ==
  ICa : Inport
  AdjCa : Inport  Port=2
  CaDiff : Sum  Inputs=+-
  CaIntegrate : Integrator
  Sum : Sum  Inputs=+-+
  a : Gain  Gain=a
  d : Gain  Gain=1/d
  f : Gain  Gain=f
  "[Ca]" : Outport
  wires:
  Sum/1 -> CaIntegrate/1
  f/1 -> Sum/1
  ICa/1 -> f/1
  a/1 -> Sum/2
  CaIntegrate/1 -> "[Ca]"/1, a/1, CaDiff/2
  AdjCa/1 -> CaDiff/1
  CaDiff/1 -> d/1
  d/1 -> Sum/3

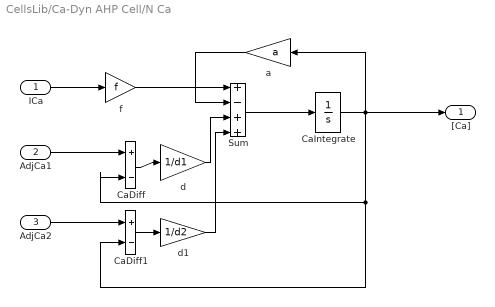
== system CellsLib/Ca-Dyn AHP Cell/N Ca ==
  ICa : Inport
  AdjCa1 : Inport  Port=2
  AdjCa2 : Inport  Port=3
  CaDiff : Sum  Inputs=+-
  CaDiff1 : Sum  Inputs=+-
  CaIntegrate : Integrator
  Sum : Sum  Inputs=+-++
  a : Gain  Gain=a
  d : Gain  Gain=1/d1
  d1 : Gain  Gain=1/d2
  f : Gain  Gain=f
  "[Ca]" : Outport
  wires:
  d/1 -> Sum/3
  CaDiff/1 -> d/1
  AdjCa1/1 -> CaDiff/1
  CaIntegrate/1 -> a/1, CaDiff/2, CaDiff1/2, "[Ca]"/1
  a/1 -> Sum/2
  ICa/1 -> f/1
  f/1 -> Sum/1
  Sum/1 -> CaIntegrate/1
  AdjCa2/1 -> CaDiff1/1
  CaDiff1/1 -> d1/1
  d1/1 -> Sum/4

== system CellsLib/Ca-Dyn AHP Cell/P Ca ==
  ICa : Inport
  AdjCa1 : Inport  Port=2
  AdjCa2 : Inport  Port=3
  CaDiff1 : Sum  Inputs=+-
  CaDiff2 : Sum  Inputs=+-
  CaIntegrate : Integrator
  Sum : Sum  Inputs=+-++
  a : Gain  Gain=a
  d1 : Gain  Gain=1/d1
  d2 : Gain  Gain=1/d2
  f : Gain  Gain=f
  "[Ca]" : Outport
  wires:
  d1/1 -> Sum/3
  CaIntegrate/1 -> a/1, "[Ca]"/1, CaDiff1/2, CaDiff2/2
  a/1 -> Sum/2
  ICa/1 -> f/1
  f/1 -> Sum/1
  Sum/1 -> CaIntegrate/1
  CaDiff1/1 -> d1/1
  AdjCa1/1 -> CaDiff1/1
  AdjCa2/1 -> CaDiff2/1
  CaDiff2/1 -> d2/1
  d2/1 -> Sum/4

== system CellsLib/Ca-Dyn AHP Cell/Slow Ca ==
  AdjCa1 : Inport
  AdjCa2 : Inport  Port=2
  AdjCa3 : Inport  Port=3
  CaDiff1 : Sum  Inputs=+-
  CaDiff2 : Sum  Inputs=+-
  CaDiff3 : Sum  Inputs=+-
  CaIntegrate : Integrator
  sum : Sum  Inputs=+++
  tdiff1 : Gain  Gain=1/tauDiff1
  tdiff2 : Gain  Gain=1/tauDiff2
  tdiff3 : Gain  Gain=1/tauDiff3
  "[Ca]" : Outport
  wires:
  AdjCa1/1 -> CaDiff1/1
  CaIntegrate/1 -> "[Ca]"/1, CaDiff1/2, CaDiff2/2, CaDiff3/2
  AdjCa2/1 -> CaDiff2/1
  AdjCa3/1 -> CaDiff3/1
  CaDiff1/1 -> tdiff1/1
  CaDiff2/1 -> tdiff2/1
  CaDiff3/1 -> tdiff3/1
  tdiff1/1 -> sum/1
  tdiff2/1 -> sum/2
  tdiff3/1 -> sum/3
  sum/1 -> CaIntegrate/1

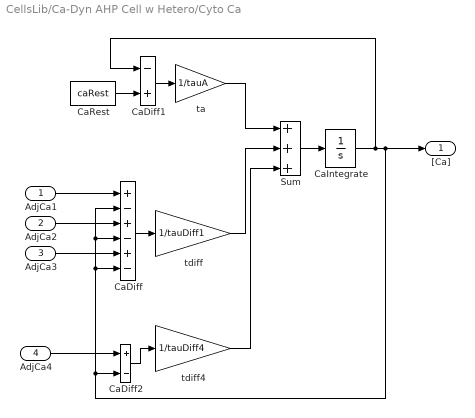
== system CellsLib/Ca-Dyn AHP Cell w Hetero/Cyto Ca ==
  AdjCa1 : Inport
  AdjCa2 : Inport  Port=2
  AdjCa3 : Inport  Port=3
  AdjCa4 : Inport  Port=4
  CaDiff : Sum  Inputs=+-+-+-
  CaDiff1 : Sum  Inputs=-+
  CaDiff2 : Sum  Inputs=+-
  CaIntegrate : Integrator  InitialCondition=caRest
  CaRest : Constant  Value=caRest
  Sum : Sum  Inputs=+++
  ta : Gain  Gain=1/tauA
  tdiff : Gain  Gain=1/tauDiff1
  tdiff4 : Gain  Gain=1/tauDiff4
  "[Ca]" : Outport
  wires:
  AdjCa4/1 -> CaDiff2/1
  tdiff4/1 -> Sum/3
  CaDiff2/1 -> tdiff4/1
  AdjCa3/1 -> CaDiff/5
  AdjCa2/1 -> CaDiff/3
  AdjCa1/1 -> CaDiff/1
  ta/1 -> Sum/1
  CaDiff1/1 -> ta/1
  CaRest/1 -> CaDiff1/2
  Sum/1 -> CaIntegrate/1
  CaIntegrate/1 -> CaDiff/2, CaDiff/4, CaDiff/6, CaDiff2/2, "[Ca]"/1, CaDiff1/1
  CaDiff/1 -> tdiff/1
  tdiff/1 -> Sum/2

== system CellsLib/Ca-Dyn AHP Cell w Hetero/L Ca ==
  ICa : Inport
  AdjCa : Inport  Port=2
  CaDiff : Sum  Inputs=+-
  CaIntegrate : Integrator
  Sum : Sum  Inputs=+-+
  a : Gain  Gain=a
  d : Gain  Gain=1/d
  f : Gain  Gain=f
  "[Ca]" : Outport
  wires:
  d/1 -> Sum/3
  CaDiff/1 -> d/1
  AdjCa/1 -> CaDiff/1
  CaIntegrate/1 -> CaDiff/2, a/1, "[Ca]"/1
  a/1 -> Sum/2
  ICa/1 -> f/1
  f/1 -> Sum/1
  Sum/1 -> CaIntegrate/1

== system CellsLib/Ca-Dyn AHP Cell w Hetero/N Ca ==
  ICa : Inport
  AdjCa1 : Inport  Port=2
  AdjCa2 : Inport  Port=3
  CaDiff : Sum  Inputs=+-
  CaDiff1 : Sum  Inputs=+-
  CaIntegrate : Integrator
  Sum : Sum  Inputs=+-++
  a : Gain  Gain=a
  d : Gain  Gain=1/d1
  d1 : Gain  Gain=1/d2
  f : Gain  Gain=f
  "[Ca]" : Outport
  wires:
  d1/1 -> Sum/4
  CaDiff1/1 -> d1/1
  AdjCa2/1 -> CaDiff1/1
  Sum/1 -> CaIntegrate/1
  f/1 -> Sum/1
  ICa/1 -> f/1
  a/1 -> Sum/2
  CaIntegrate/1 -> "[Ca]"/1, CaDiff1/2, CaDiff/2, a/1
  AdjCa1/1 -> CaDiff/1
  CaDiff/1 -> d/1
  d/1 -> Sum/3

== system CellsLib/Ca-Dyn AHP Cell w Hetero/P Ca ==
  ICa : Inport
  AdjCa1 : Inport  Port=2
  AdjCa2 : Inport  Port=3
  CaDiff1 : Sum  Inputs=+-
  CaDiff2 : Sum  Inputs=+-
  CaIntegrate : Integrator
  Sum : Sum  Inputs=+-++
  a : Gain  Gain=a
  d1 : Gain  Gain=1/d1
  d2 : Gain  Gain=1/d2
  f : Gain  Gain=f
  "[Ca]" : Outport
  wires:
  d2/1 -> Sum/4
  CaDiff2/1 -> d2/1
  AdjCa2/1 -> CaDiff2/1
  AdjCa1/1 -> CaDiff1/1
  CaDiff1/1 -> d1/1
  Sum/1 -> CaIntegrate/1
  f/1 -> Sum/1
  ICa/1 -> f/1
  a/1 -> Sum/2
  CaIntegrate/1 -> CaDiff2/2, CaDiff1/2, "[Ca]"/1, a/1
  d1/1 -> Sum/3

== system CellsLib/Ca-Dyn AHP Cell w Hetero/Slow Ca ==
  AdjCa1 : Inport
  AdjCa2 : Inport  Port=2
  AdjCa3 : Inport  Port=3
  CaDiff1 : Sum  Inputs=+-
  CaDiff2 : Sum  Inputs=+-
  CaDiff3 : Sum  Inputs=+-
  CaIntegrate : Integrator
  sum : Sum  Inputs=+++
  tdiff1 : Gain  Gain=1/tauDiff1
  tdiff2 : Gain  Gain=1/tauDiff2
  tdiff3 : Gain  Gain=1/tauDiff3
  "[Ca]" : Outport
  wires:
  sum/1 -> CaIntegrate/1
  tdiff3/1 -> sum/3
  tdiff2/1 -> sum/2
  tdiff1/1 -> sum/1
  CaDiff3/1 -> tdiff3/1
  CaDiff2/1 -> tdiff2/1
  CaDiff1/1 -> tdiff1/1
  AdjCa3/1 -> CaDiff3/1
  AdjCa2/1 -> CaDiff2/1
  CaIntegrate/1 -> CaDiff3/2, CaDiff2/2, CaDiff1/2, "[Ca]"/1
  AdjCa1/1 -> CaDiff1/1

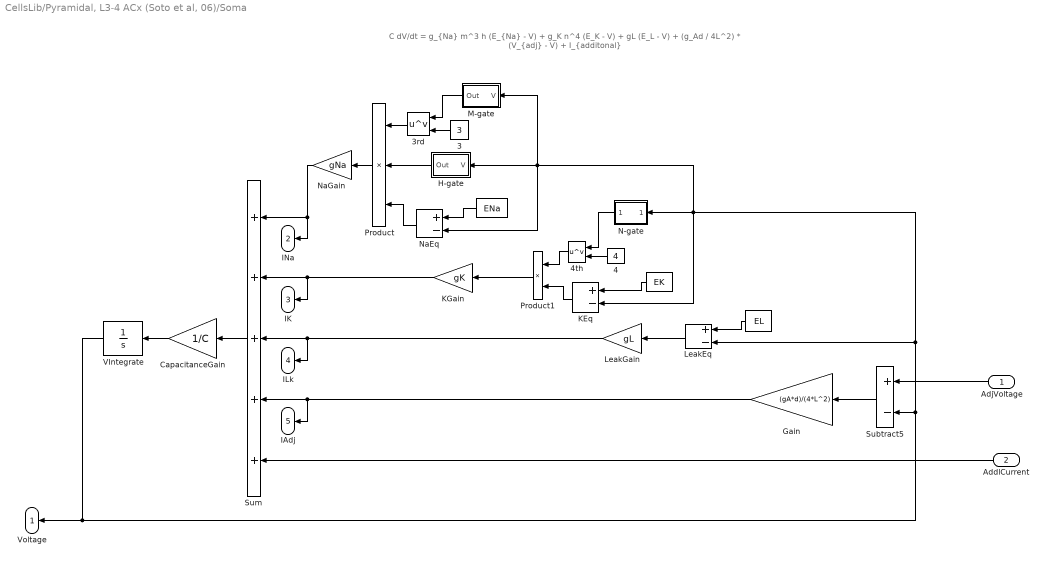
== system CellsLib/Pyramidal, L3-4 ACx (Soto et al, 06)/Soma ==
  note: C dV/dt = g_{Na} m^3 h (E_{Na} - V) + g_K n^4 (E_K - V) + gL (E_L - V) + (g_Ad / 4L^2) * (V_{adj} - V) + I_{additonal}
  AdjVoltage : Inport
  AddlCurrent : Inport  Port=2
  " " : Constant  Value=EL
  "  " : Constant  Value=ENa
  "   " : Constant  Value=EK
  " 3" : Constant  Value=3
  3rd : Math  Operator=pow  SaturateOnIntegerOverflow=on
  4 : Constant  Value=4
  4th : Math  Operator=pow  SaturateOnIntegerOverflow=on
  CapacitanceGain : Gain  Gain=1/C
  Gain : Gain  Gain=(gA*d)/(4*L^2)
  H-gate : Subsystem
  KEq : Sum  Inputs=+-
  KGain : Gain  Gain=gK
  LeakEq : Sum  Inputs=+-
  LeakGain : Gain  Gain=gL
  M-gate : Subsystem
  N-gate : Subsystem
  NaEq : Sum  Inputs=+-
  NaGain : Gain  Gain=gNa
  Product : Product  Inputs=3  RndMeth=Zero
  Product1 : Product  RndMeth=Zero
  Subtract5 : Sum  Inputs=+-
  Sum : Sum  Inputs=+++++
  VIntegrate : Integrator  InitialCondition=V0
  Voltage : Outport
  INa : Outport  Port=2
  IK : Outport  Port=3
  ILk : Outport  Port=4
  IAdj : Outport  Port=5
  wires:
  AdjVoltage/1 -> Subtract5/1
  Subtract5/1 -> Gain/1
  LeakGain/1 -> ILk/1, Sum/3
  LeakEq/1 -> LeakGain/1
  " "/1 -> LeakEq/1
  Sum/1 -> CapacitanceGain/1
  CapacitanceGain/1 -> VIntegrate/1
  VIntegrate/1 -> Subtract5/2, LeakEq/2, N-gate/1(In1), KEq/2, H-gate/1(V), M-gate/1(V), NaEq/2, Voltage/1
  AddlCurrent/1 -> Sum/5
  Gain/1 -> IAdj/1, Sum/4
  4/1 -> 4th/2
  N-gate/1(Out1) -> 4th/1
  " 3"/1 -> 3rd/2
  M-gate/1(Out) -> 3rd/1
  3rd/1 -> Product/1
  H-gate/1(Out) -> Product/2
  "   "/1 -> KEq/1
  NaEq/1 -> Product/3
  Product/1 -> NaGain/1
  Product1/1 -> KGain/1
  NaGain/1 -> INa/1, Sum/1
  KGain/1 -> IK/1, Sum/2
  4th/1 -> Product1/1
  KEq/1 -> Product1/2
  "  "/1 -> NaEq/1

== system CellsLib/Pyramidal, L3-4 ACx (Soto et al, 06)/Soma/H-gate ==
  V : Inport
  1 : Constant
  Add : Sum  Inputs=-+
  Integrator : Integrator  InitialCondition=1
  Product : Product  RndMeth=Zero
  Product1 : Product  RndMeth=Zero
  Subtract : Sum  Inputs=+-
  alphaH : MATLABFcn  MATLABFcn=0.128 * exp( -(50+u) / 18)
  betaH : MATLABFcn  MATLABFcn=4 ./ (exp(- (27+u)/5 ) + 1)
  Out : Outport
  wires:
  Add/1 -> Integrator/1
  Integrator/1 -> Subtract/2, Out/1, Product1/1
  1/1 -> Subtract/1
  Subtract/1 -> Product/2
  Product/1 -> Add/2
  alphaH/1 -> Product/1
  V/1 -> betaH/1, alphaH/1
  Product1/1 -> Add/1
  betaH/1 -> Product1/2

== system CellsLib/Pyramidal, L3-4 ACx (Soto et al, 06)/Soma/M-gate ==
  V : Inport
  1 : Constant
  Add : Sum  Inputs=-+
  Integrator : Integrator
  Product : Product  RndMeth=Zero
  Product1 : Product  RndMeth=Zero
  Subtract : Sum  Inputs=+-
  alphaM : MATLABFcn  MATLABFcn=0.32 .* (50+u) ./ (1-exp(-(50+u) ./ 4 ))
  betaM : MATLABFcn  MATLABFcn=0.28 .* (27+u) ./ (exp( (27+u) ./5 ) - 1)
  Out : Outport
  wires:
  Add/1 -> Integrator/1
  Integrator/1 -> Subtract/2, Out/1, Product1/1
  1/1 -> Subtract/1
  Subtract/1 -> Product/2
  Product/1 -> Add/2
  V/1 -> betaM/1, alphaM/1
  alphaM/1 -> Product/1
  Product1/1 -> Add/1
  betaM/1 -> Product1/2

== system CellsLib/Pyramidal, L3-4 ACx (Soto et al, 06)/Soma/N-gate ==
  In1 : Inport
  Add : Sum  Inputs=-+
  Constant : Constant
  Integrator : Integrator
  Product : Product  RndMeth=Zero
  Product1 : Product  RndMeth=Zero
  Subtract : Sum  Inputs=+-
  alphaN : MATLABFcn  MATLABFcn=0.032 .* (52+u) ./ (1 - exp( -(52+u) ./ 5 ) )
  betaN : MATLABFcn  MATLABFcn=0.5 .* exp(-(57+u) ./ 40)
  Out1 : Outport
  wires:
  betaN/1 -> Product1/2
  Add/1 -> Integrator/1
  Integrator/1 -> Subtract/2, Out1/1, Product1/1
  Constant/1 -> Subtract/1
  Subtract/1 -> Product/2
  Product/1 -> Add/2
  Product1/1 -> Add/1
  In1/1 -> alphaN/1, betaN/1
  alphaN/1 -> Product/1
